simulink model "rtwdemo_slcustcode"  (Simulink 6.0)
settings: Solver=FixedStepDiscrete  StartTime=0.0  StopTime=48  FixedStep=1  RelTol=1e-3
libraries: rtwdemowidgets x3
settings Model: CovMetricSettings=d  Creator=The MathWorks Inc.  LastModifiedBy=batserve  ParamWorkspaceSource=ReferencedWorkspace  ExtModeTrigMode=oneshot  ExtModeArmWhenConnect=off  ExtModeAutoUpdateStatusClock=off
settings DataIOCC: LimitDataPoints=off  SaveFormat=StructureWithTime  SaveOutput=off  SaveTime=off  SignalLoggingName=sigsOut
settings OptimizationCC: InlineParams=on  EnforceIntegerDowncast=off  StateBitsets=on  DataBitsets=on  UseTempVars=on
settings DebuggingCC: CheckExecutionContextPreStartOutputMsg=on  CheckExecutionContextRuntimeOutputMsg=on  SolverPrmCheckMsg=none  IntegerOverflowMsg=none
settings ModelReferenceCC: UpdateModelReferenceTargets=IfOutOfDate
settings RTWCC: TLCOptions=-p0 -aWarnNonSaturatedBlocks=0  GenerateReport=on  RTWVerbose=off  ProcessScript=grt_make_rtw_hook  LaunchReport=on
settings RTWCC: CustomSourceCode=|
  | /* Declared from Configration Parameters RTW Custom Code Page (Source file) */
  | int_T GLOBAL_INT2 = -1;
settings RTWCC: CustomInitializer=|
  | /* Declared from Configuration Parameters RTW Custom Code Page (Initialize function) */
  | GLOBAL_INT2 = 1;
settings CodeAppCC: ForceParamTrailComments=on  PrefixModelToSubsysFcnNames=off
settings GRTTargetCC: MatFileLogging=off

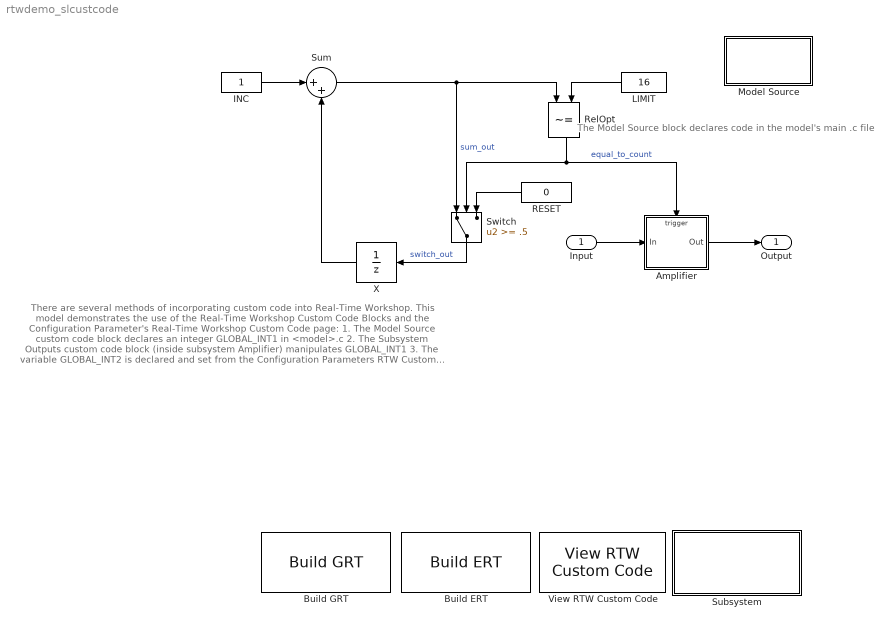
== system rtwdemo_slcustcode ==
  note: There are several methods of incorporating custom code into Real-Time Workshop.  This model
      | demonstrates the use of the Real-Time Workshop Custom Code Blocks and the Configuration
      | Parameter's Real-Time Workshop Custom Code page:
      |
      | 1. The Model Source custom code block declares an integer GLOBAL_INT1 in <model>.c
      | 2. The Subsystem Outputs custom code block (inside subsystem Amplifier) manipulates GLOBAL_INT1
      | 3. The variable GLOBAL_INT2 is declared and set from the Configuration Parameters RTW Custom
      |     Code page, from the "Source file" and "Initialize function," respectively.
      |
      | There is some overlap between custom code blocks and custom code via the configuration parameters,
      | but overall the custom code blocks provide much finer granularity of code placement, and they
      | are graphical.
  note: The Model Source block
      | declares code in the
      | model's main .c file
  Input : Inport  Port=1  DataType=int32  LatchInput=off
  Amplifier : Subsystem  TreatAsAtomicUnit=on  PropExecContextAcrossSSBoundary=on
  Build ERT : rtwdemowidgets/Build ERT  attrib_overrides={}
  Build GRT : rtwdemowidgets/Build GRT  attrib_overrides={}
  INC : Constant
  LIMIT : Constant  Orientation=left  Value=16
  Model Source : Subsystem  PropExecContextAcrossSSBoundary=on
      settings: CopyFcn=cccopyfcn(gcb)  OpenFcn=ccopenfcn('Model Source')
      mask Type: Model Source
      mask Description: Add code to the model .c file
      mask Help: This source file block contains text fields to insert custom user code at the top and bottom of model.c file.
      mask Display: disp('Model\nSource');
  RESET : Constant  Orientation=left  Value=0
  RelOpt : RelationalOperator  Orientation=down  Operator=~=  InputSameDT=on
  Subsystem : Subsystem  PropExecContextAcrossSSBoundary=on
      settings: OpenFcn=custcode
      mask Display:
      | disp(['View Custom\nCode ',...
      | 	  'Library\n(double-click)'])
  Sum : Sum  Inputs=|++  InputSameDT=on
  Switch : Switch  Orientation=down  Threshold=.5  SaturateOnIntegerOverflow=on  InputSameDT=on
  View RTW Custom Code : rtwdemowidgets/View RTW Custom Code
  X : UnitDelay  Orientation=left  StateIdentifier=X
  Output : Outport
  wires:
  INC/1 -> Sum/1
  X/1 -> Sum/2
  Switch/1 -> X/1  "switch_out"
  Sum/1 -> Switch/1, RelOpt/1  "sum_out"
  LIMIT/1 -> RelOpt/2
  Input/1 -> Amplifier/1(In)
  RESET/1 -> Switch/3
  RelOpt/1 -> Switch/2, Amplifier/Trigger  "equal_to_count"
  Amplifier/1(Out) -> Output/1

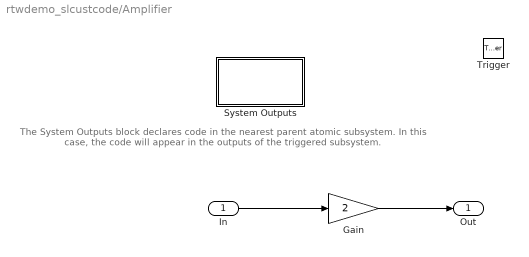
== system rtwdemo_slcustcode/Amplifier ==
  note: The System Outputs block declares code in the nearest
      | parent atomic subsystem.  In this case, the code will
      | appear in the outputs of the triggered subsystem.
  In : Inport  Port=1  LatchInput=off
  Trigger : TriggerPort
  Gain : Gain  Gain=2
  System Outputs : Subsystem  PropExecContextAcrossSSBoundary=on
      settings: CopyFcn=cccopyfcn(gcb)  OpenFcn=ccopenfcn('System Outputs Function')
      mask Type: System Outputs
      mask Description: Add code to a systems Outputs function
      mask Help: This block contains text fields to insert custom user code sections at the declaration, execution and exit sections of the systems outputs function.  By placing this block inside a subsytem, the custom user code will appear in that subsystems function.
      mask Display: disp('System\nOutputs');
  Out : Outport  InitialOutput=0
  wires:
  In/1 -> Gain/1
  Gain/1 -> Out/1

== system rtwdemo_slcustcode/Model Source ==

== system rtwdemo_slcustcode/Subsystem ==

== system rtwdemo_slcustcode/Amplifier/System Outputs ==
